simulink model "ProposedProblem1"  (R2013a)
settings: Solver=ode45  StartTime=0.0  StopTime=720000  RelTol=1e-3
undefined symbols (not defined in the file): des, gcbh
settings Model: Creator=gabig  LastModifiedBy=gabig

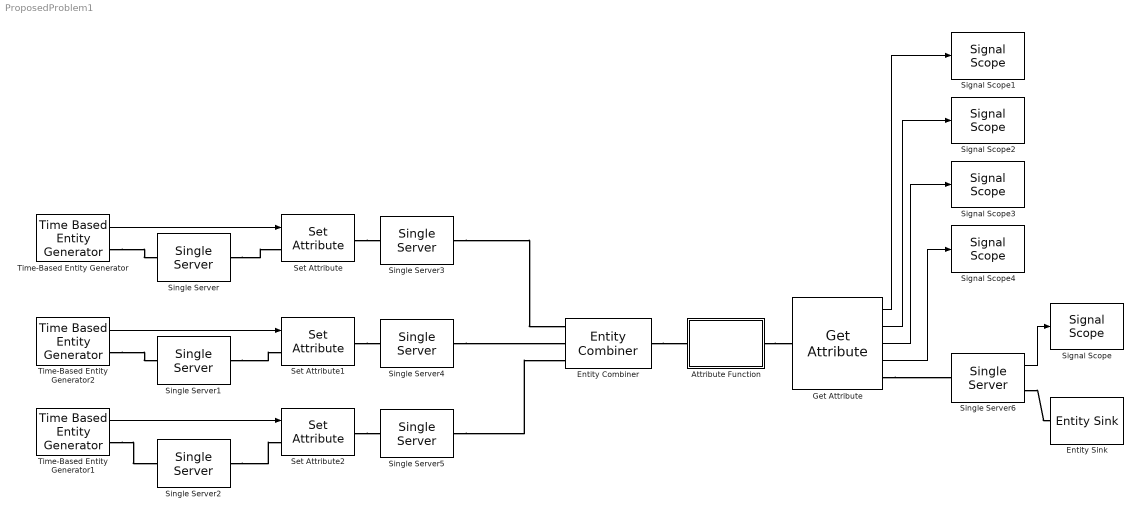
== system ProposedProblem1 ==
  Attribute Function : Subsystem  LoadFcn=des.afb.attributefunction_support(gcb,'LoadFcn');  StartFcn=des.afb.attributefunction_support(gcb,'StartFcn');  mask(Attribute Function){OutputNamePrefix=out_}
      mask prompts: OutputNamePrefix "Prefix name"
      settings: CopyFcn=des.afb.attributefunction_support(gcb,'CopyFcn');  OpenFcn=des.afb.attributefunction_support(gcb,'OpenFcn');  ErrorFcn=des.afb.error_redirect
      mask Help: slhelp(gcbh)
      mask Display: image(des_iconLoad('attribFunction.jpg'),'center');
  Entity Combiner : EntityCombiner
  Entity Sink : EntitySink
  Get Attribute : GetAttribute  AttributeName=AutoNumber|Chassis|Engine|Transmission  AttributeMissing=Error|Error|Error|Error  AttributeDefaultValue=1|1|1|1  AttributeTreatAsVector=1|1|1|1  AttributeSendTiming=After entity departure|After entity departure|After entity departure|After entity departure  EvaluatedDefaultAttributeValue={ [];[];[];[]}
      settings: OutputPortMap=o1,o2,o3,o4
  Set Attribute : SetAttribute  AttributeName=Engine  AttributeFrom=Signal port  EvaluatedAttributeValue={ []}
  Set Attribute1 : SetAttribute  AttributeName=Chassis  AttributeFrom=Signal port  EvaluatedAttributeValue={ []}
  Set Attribute2 : SetAttribute  AttributeName=Transmission  AttributeFrom=Signal port  EvaluatedAttributeValue={ []}
  Signal Scope{,1..4} (5 alike) : SignalScope  LoadFcn=des.scope.CallbackSupport('seLoadFcn',gcbh)  StartFcn=des.scope.CallbackSupport('seStartFcn',gcbh)  StopFcn=des.scope.CallbackSupport('seStopFcn',gcbh)
      settings: CopyFcn=des.scope.CallbackSupport('seCopyFcn',gcbh)  DeleteFcn=des.scope.CallbackSupport('seDeleteFcn',gcbh)  PreSaveFcn=des.scope.CallbackSupport('sePreSaveFcn',gcbh)  NameChangeFcn=des.scope.CallbackSupport('seNameChangeFcn',gcbh)  OpenFcn=des.scope.CallbackSupport('seOpenFcn',gcbh)
  Single Server : SingleServer  ServiceTime=0
  Single Server1 : SingleServer  ServiceTime=0
  Single Server2 : SingleServer  ServiceTime=0
  Single Server3 : SingleServer  ServiceTime=2160
  Single Server4 : SingleServer  ServiceTime=1440
  Single Server5 : SingleServer  ServiceTime=1440
  Single Server6 : SingleServer  ServiceTime=1080  StatNumberDeparted=on
  Time-Based Entity Generator : TimeBasedEntityGenerator  Period=2880  StatNumberDeparted=on
  Time-Based Entity Generator1 : TimeBasedEntityGenerator  Period=2160  StatNumberDeparted=on
  Time-Based Entity Generator2 : TimeBasedEntityGenerator  Period=1440  StatNumberDeparted=on
  wires:
  Time-Based Entity Generator1/1 -> Set Attribute2/1
  Time-Based Entity Generator2/1 -> Set Attribute1/1
  Time-Based Entity Generator/1 -> Set Attribute/1
  Single Server6/1 -> Signal Scope/1
  Get Attribute/1 -> Signal Scope1/1
  Get Attribute/2 -> Signal Scope2/1
  Get Attribute/3 -> Signal Scope3/1
  Get Attribute/4 -> Signal Scope4/1
  connections:
  Single Server4/RConn1 -- Entity Combiner/LConn2
  Single Server1/RConn1 -- Set Attribute1/LConn1
  Set Attribute1/RConn1 -- Single Server4/LConn1
  Set Attribute/RConn1 -- Single Server3/LConn1
  Time-Based Entity Generator1/RConn1 -- Single Server2/LConn1
  Single Server2/RConn1 -- Set Attribute2/LConn1
  Set Attribute2/RConn1 -- Single Server5/LConn1
  Single Server6/RConn1 -- Entity Sink/LConn1
  Single Server/RConn1 -- Set Attribute/LConn1
  Single Server3/RConn1 -- Entity Combiner/LConn1
  Single Server5/RConn1 -- Entity Combiner/LConn3
  Time-Based Entity Generator/RConn1 -- Single Server/LConn1
  Time-Based Entity Generator2/RConn1 -- Single Server1/LConn1
  Entity Combiner/RConn1 -- Attribute Function/LConn1
  Attribute Function/RConn1 -- Get Attribute/LConn1
  Get Attribute/RConn1 -- Single Server6/LConn1

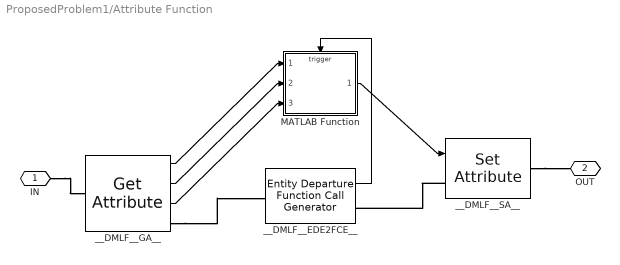
== system ProposedProblem1/Attribute Function ==
  MATLAB Function : MATLAB Function  TreatAsAtomicUnit=on
  __DMLF__EDE2FCE__ : EntityDepartureFunctionCallGenerator  TimingFunctionCallF1=Before entity departure  IsInsideAFB=on
  __DMLF__GA__ : GetAttribute  AttributeName=Engine|Chassis|Transmission  AttributeMissing=Error|Error|Error  AttributeDefaultValue=1|1|1  AttributeTreatAsVector=1|1|1  AttributeSendTiming=Before entity departure|Before entity departure|Before entity departure  EvaluatedDefaultAttributeValue={ [];[];[]}  IsInsideAFB=on
      settings: OutputPortMap=o1,o2,o3
  __DMLF__SA__ : SetAttribute  AttributeName=AutoNumber  AttributeFrom=Signal port  EvaluatedAttributeValue={ []}  IsInsideAFB=on
  IN : PMIOPort  Port=1  Side=Left
  OUT : PMIOPort  Port=2  Side=Right
  wires:
  __DMLF__EDE2FCE__/1 -> MATLAB Function/Trigger
  __DMLF__GA__/1 -> MATLAB Function/1(Engine)
  __DMLF__GA__/2 -> MATLAB Function/2(Chassis)
  __DMLF__GA__/3 -> MATLAB Function/3(Transmission)
  MATLAB Function/1(out_AutoNumber) -> __DMLF__SA__/1
  connections:
  __DMLF__SA__/LConn1 -- __DMLF__EDE2FCE__/RConn1
  __DMLF__GA__/RConn1 -- __DMLF__EDE2FCE__/LConn1
  IN/RConn1 -- __DMLF__GA__/LConn1
  __DMLF__SA__/RConn1 -- OUT/RConn1

== matlab function ProposedProblem1/Attribute Function/MATLAB Function ==
  data: Engine input; out_AutoNumber output; Chassis input; Transmission input
  events: trigger input FUNCTION_CALL_EVENT
function out_AutoNumber = fcn(Engine, Chassis, Transmission)
%FCN    Access and modify attributes with MATLAB 
% 
% Input arguments must match the attribute names.
% Output arguments must be out_<AttributeName>,
% e.g., out_ServiceTime where ServiceTime is the attribute name.
% 
% The output attribute will be created if it is not present.
%

out_AutoNumber = Engine + 10 * Transmission + 100 * Chassis;
